simulink model "ZSM_TeslaModelS_statKreisfahrt"  (R2020b)
settings: Solver=FixedStepDiscrete  StartTime=0.0  StopTime=simtime  FixedStep=stepsize  RelTol=1e-3
undefined symbols (not defined in the file): activate_stop, activate_stop_vmax, ay_stop, ayObs, ayStiff, Bat_param, deltav_ist, DiscIntNeverNeededParam, EG_wunsch, magnitude, mu_road_LF, mu_road_LR, mu_road_RF, mu_road_RR, par_ASR, par_MDT, par_TIR, par_VEH, select_delta_h, select_M_wheel, stepsize, t, temp_betriebsstrategie, temperature_LTrange, track_left, track_right
libraries: Library_ASK x36, simulink x16, pid_lib x2, dspstat3 x2, Library_Betriebsstrategie x2, vehicle_model x2, pacejka_trans x1
(part 5 of 7)

== system ZSM_TeslaModelS_statKreisfahrt/Vehicle/Betriebsstrategie/Momentenverteilung_und_Schaltstrategie1/Limitierungen gesamt (mit MVS Limits)/Aktuatoren und Delta TV ==
  Aktuator : Constant  Value=par_MDT.AUS.akt.OD_VA
  Aktuator1 : Constant  Value=0
  Aktuator10 : Constant  Value=par_MDT.AUS.akt.TS_VA
  Aktuator11 : Constant  Value=par_MDT.AUS.akt.TS_HA
  Aktuator3 : Constant  Value=par_MDT.AUS.akt.eTV_VA
  Aktuator4 : Constant  Value=par_MDT.AUS.akt.az_VA
  Aktuator5 : Constant  Value=par_MDT.AUS.akt.OD_HA
  Aktuator6 : Constant  Value=0
  Aktuator8 : Constant  Value=par_MDT.AUS.akt.eTV_HA
  Aktuator9 : Constant  Value=par_MDT.AUS.akt.az_HA
  Limit elektrisches Überlagerungsgetriebe : Constant  Value=595
  Limit mechanisches Überlagerungsgetriebe1 : Constant  Value=595
  Limit mechanisches Überlagerungsgetriebe2 : Constant  Value=595
  Limit mechanisches Überlagerungsgetriebe3 : Constant  Value=595
  Logical Operator : Logic  Operator=NOT  AllPortsSameDT=off  OutDataTypeStr=boolean
  Logical Operator1 : Logic  Operator=NOT  AllPortsSameDT=off  OutDataTypeStr=boolean
  TV Moment pro Achse : MATLAB Function  TreatAsAtomicUnit=on
  Zuweisung Aktuatoren : MATLAB Function  TreatAsAtomicUnit=on
  Delta_T_f : Outport  VectorParamsAs1DForOutWhenUnconnected=off
  Delta_T_r : Outport  Port=2  VectorParamsAs1DForOutWhenUnconnected=off
  A_f : Outport  Port=3  VectorParamsAs1DForOutWhenUnconnected=off
  A_r : Outport  Port=4  VectorParamsAs1DForOutWhenUnconnected=off
  wires:
  Zuweisung Aktuatoren/1(a_f) -> A_f/1, TV Moment pro Achse/6(a_f)
  Aktuator9/1 -> Logical Operator1/1
  Aktuator8/1 -> Zuweisung Aktuatoren/9(A9)
  Aktuator11/1 -> Zuweisung Aktuatoren/8(A8)
  Aktuator6/1 -> Zuweisung Aktuatoren/7(A7)
  Aktuator5/1 -> Zuweisung Aktuatoren/6(A6)
  Aktuator4/1 -> Logical Operator/1
  Aktuator3/1 -> Zuweisung Aktuatoren/4(A4)
  Aktuator10/1 -> Zuweisung Aktuatoren/3(A3)
  Aktuator1/1 -> Zuweisung Aktuatoren/2(A2)
  Aktuator/1 -> Zuweisung Aktuatoren/1(A1)
  Zuweisung Aktuatoren/2(a_r) -> A_r/1, TV Moment pro Achse/7(a_r)
  TV Moment pro Achse/1(Delta_T_f) -> Delta_T_f/1
  TV Moment pro Achse/2(Delta_T_r) -> Delta_T_r/1
  Limit elektrisches Überlagerungsgetriebe/1 -> TV Moment pro Achse/1(L1)
  Limit mechanisches Überlagerungsgetriebe1/1 -> TV Moment pro Achse/2(L2)
  Limit mechanisches Überlagerungsgetriebe2/1 -> TV Moment pro Achse/3(L3)
  Limit mechanisches Überlagerungsgetriebe3/1 -> TV Moment pro Achse/4(L4)
  Logical Operator/1 -> Zuweisung Aktuatoren/5(A5)
  Logical Operator1/1 -> Zuweisung Aktuatoren/10(A10)

== system ZSM_TeslaModelS_statKreisfahrt/Vehicle/Betriebsstrategie/Momentenverteilung_und_Schaltstrategie1/Motor Limits/Limit_F_lb ==
  Raddrehzahl : Inport
  Drehmoment : Product
  Drehzahl : Product
  Getriebeuebersetzung : Constant  Value=par_MDT.VA.trans.i_gears
  Getriebewirkungsgrad : Constant  Value=par_MDT.VA.trans.wkg
  M_Reku : Lookup_n-D  NumberOfTableDimensions=1  BreakpointsForDimension1=par_MDT.VA.em.MaxGeneratorTrqCurve_w  Table=par_MDT.VA.em.MaxGeneratorTrqCurve_M  ExtrapMethod=Clip  UseLastTableValue=on  InternalRulePriority=Speed  RndMeth=Simplest  InputSameDT=on
  MinMax : MinMax  Function=max
  Rueckrechnung : Product
  Moment : Outport  VectorParamsAs1DForOutWhenUnconnected=off
  wires:
  Drehzahl/1 -> M_Reku/1
  Getriebeuebersetzung/1 -> Drehzahl/2, Drehmoment/2
  Raddrehzahl/1 -> Drehzahl/1
  M_Reku/1 -> Drehmoment/1
  Drehmoment/1 -> Rueckrechnung/1
  Rueckrechnung/1 -> MinMax/1
  Getriebewirkungsgrad/1 -> Rueckrechnung/2
  MinMax/1 -> Moment/1

== system ZSM_TeslaModelS_statKreisfahrt/Vehicle/Betriebsstrategie/Momentenverteilung_und_Schaltstrategie1/Motor Limits/Limit_F_ub ==
  Raddrehzahl : Inport
  Drehmoment : Product
  Drehzahl : Product
  Getriebeuebersetzung : Constant  Value=par_MDT.VA.trans.i_gears
  Getriebewirkungsgrad : Constant  Value=par_MDT.VA.trans.wkg
  M_Antr : Lookup_n-D  NumberOfTableDimensions=1  BreakpointsForDimension1=par_MDT.VA.em.MaxMotorTrqCurve_w  Table=par_MDT.VA.em.MaxMotorTrqCurve_M  ExtrapMethod=Clip  UseLastTableValue=on  InternalRulePriority=Speed  RndMeth=Simplest  InputSameDT=on
  MinMax : MinMax  Function=max
  Rueckrechnung : Product
  Moment : Outport  VectorParamsAs1DForOutWhenUnconnected=off
  wires:
  Drehzahl/1 -> M_Antr/1
  Getriebeuebersetzung/1 -> Drehzahl/2, Drehmoment/2
  Raddrehzahl/1 -> Drehzahl/1
  M_Antr/1 -> Drehmoment/1
  Drehmoment/1 -> Rueckrechnung/1
  Rueckrechnung/1 -> MinMax/1
  Getriebewirkungsgrad/1 -> Rueckrechnung/2
  MinMax/1 -> Moment/1

== system ZSM_TeslaModelS_statKreisfahrt/Vehicle/Betriebsstrategie/Momentenverteilung_und_Schaltstrategie1/Motor Limits/Limit_LF_lb ==
  Raddrehzahl : Inport
  Drehmoment : Product
  Drehzahl : Product
  Getriebeuebersetzung : Constant  Value=par_MDT.VA.trans.i_gears
  Getriebewirkungsgrad : Constant  Value=par_MDT.VA.trans.wkg
  M_Reku : Lookup_n-D  NumberOfTableDimensions=1  BreakpointsForDimension1=par_MDT.VA.em.MaxGeneratorTrqCurve_w  Table=par_MDT.VA.em.MaxGeneratorTrqCurve_M  ExtrapMethod=Clip  UseLastTableValue=on  InternalRulePriority=Speed  RndMeth=Simplest  InputSameDT=on
  MinMax : MinMax  Function=max
  Rueckrechnung : Product
  Moment : Outport  VectorParamsAs1DForOutWhenUnconnected=off
  wires:
  Drehzahl/1 -> M_Reku/1
  Getriebeuebersetzung/1 -> Drehzahl/2, Drehmoment/2
  Raddrehzahl/1 -> Drehzahl/1
  M_Reku/1 -> Drehmoment/1
  Drehmoment/1 -> Rueckrechnung/1
  Rueckrechnung/1 -> MinMax/1
  Getriebewirkungsgrad/1 -> Rueckrechnung/2
  MinMax/1 -> Moment/1

== system ZSM_TeslaModelS_statKreisfahrt/Vehicle/Betriebsstrategie/Momentenverteilung_und_Schaltstrategie1/Motor Limits/Limit_LF_ub ==
  Raddrehzahl : Inport
  Drehmoment : Product
  Drehzahl : Product
  Getriebeuebersetzung : Constant  Value=par_MDT.VA.trans.i_gears
  Getriebewirkungsgrad : Constant  Value=par_MDT.VA.trans.wkg
  M_Antr : Lookup_n-D  NumberOfTableDimensions=1  BreakpointsForDimension1=par_MDT.VA.em.MaxMotorTrqCurve_w  Table=par_MDT.VA.em.MaxMotorTrqCurve_M  ExtrapMethod=Clip  UseLastTableValue=on  InternalRulePriority=Speed  RndMeth=Simplest  InputSameDT=on
  MinMax : MinMax  Function=max
  Rueckrechnung : Product
  Moment : Outport  VectorParamsAs1DForOutWhenUnconnected=off
  wires:
  Drehzahl/1 -> M_Antr/1
  Getriebeuebersetzung/1 -> Drehzahl/2, Drehmoment/2
  Raddrehzahl/1 -> Drehzahl/1
  M_Antr/1 -> Drehmoment/1
  Drehmoment/1 -> Rueckrechnung/1
  Rueckrechnung/1 -> MinMax/1
  Getriebewirkungsgrad/1 -> Rueckrechnung/2
  MinMax/1 -> Moment/1

== system ZSM_TeslaModelS_statKreisfahrt/Vehicle/Betriebsstrategie/Momentenverteilung_und_Schaltstrategie1/Motor Limits/Limit_LR_lb ==
  Raddrehzahl : Inport
  Drehmoment : Product
  Drehzahl : Product
  Getriebeuebersetzung : Constant  Value=par_MDT.HA.trans.i_gears
  Getriebewirkungsgrad : Constant  Value=par_MDT.HA.trans.wkg
  M_Reku : Lookup_n-D  NumberOfTableDimensions=1  BreakpointsForDimension1=par_MDT.HA.em.MaxGeneratorTrqCurve_w  Table=par_MDT.HA.em.MaxGeneratorTrqCurve_M  ExtrapMethod=Clip  UseLastTableValue=on  InternalRulePriority=Speed  RndMeth=Simplest  InputSameDT=on
  MinMax : MinMax  Function=max
  Rueckrechnung : Product
  Moment : Outport  VectorParamsAs1DForOutWhenUnconnected=off
  wires:
  Drehzahl/1 -> M_Reku/1
  Getriebeuebersetzung/1 -> Drehzahl/2, Drehmoment/2
  Raddrehzahl/1 -> Drehzahl/1
  M_Reku/1 -> Drehmoment/1
  Drehmoment/1 -> Rueckrechnung/1
  Rueckrechnung/1 -> MinMax/1
  Getriebewirkungsgrad/1 -> Rueckrechnung/2
  MinMax/1 -> Moment/1

== system ZSM_TeslaModelS_statKreisfahrt/Vehicle/Betriebsstrategie/Momentenverteilung_und_Schaltstrategie1/Motor Limits/Limit_LR_ub ==
  Raddrehzahl : Inport
  Drehmoment : Product
  Drehzahl : Product
  Getriebeuebersetzung : Constant  Value=par_MDT.HA.trans.i_gears
  Getriebewirkungsgrad : Constant  Value=par_MDT.HA.trans.wkg
  M_Antr : Lookup_n-D  NumberOfTableDimensions=1  BreakpointsForDimension1=par_MDT.HA.em.MaxMotorTrqCurve_w  Table=par_MDT.HA.em.MaxMotorTrqCurve_M  ExtrapMethod=Clip  UseLastTableValue=on  InternalRulePriority=Speed  RndMeth=Simplest  InputSameDT=on
  MinMax : MinMax  Function=max
  Rueckrechnung : Product
  Moment : Outport  VectorParamsAs1DForOutWhenUnconnected=off
  wires:
  Drehzahl/1 -> M_Antr/1
  Getriebeuebersetzung/1 -> Drehzahl/2, Drehmoment/2
  Raddrehzahl/1 -> Drehzahl/1
  M_Antr/1 -> Drehmoment/1
  Drehmoment/1 -> Rueckrechnung/1
  Rueckrechnung/1 -> MinMax/1
  Getriebewirkungsgrad/1 -> Rueckrechnung/2
  MinMax/1 -> Moment/1

== system ZSM_TeslaModelS_statKreisfahrt/Vehicle/Betriebsstrategie/Momentenverteilung_und_Schaltstrategie1/Motor Limits/Limit_RF_lb ==
  Raddrehzahl : Inport
  Drehmoment : Product
  Drehzahl : Product
  Getriebeuebersetzung : Constant  Value=par_MDT.VA.trans.i_gears
  Getriebewirkungsgrad : Constant  Value=par_MDT.VA.trans.wkg
  M_Reku : Lookup_n-D  NumberOfTableDimensions=1  BreakpointsForDimension1=par_MDT.VA.em.MaxGeneratorTrqCurve_w  Table=par_MDT.VA.em.MaxGeneratorTrqCurve_M  ExtrapMethod=Clip  UseLastTableValue=on  InternalRulePriority=Speed  RndMeth=Simplest  InputSameDT=on
  MinMax : MinMax  Function=max
  Rueckrechnung : Product
  Moment : Outport  VectorParamsAs1DForOutWhenUnconnected=off
  wires:
  Drehzahl/1 -> M_Reku/1
  Getriebeuebersetzung/1 -> Drehzahl/2, Drehmoment/2
  Raddrehzahl/1 -> Drehzahl/1
  M_Reku/1 -> Drehmoment/1
  Drehmoment/1 -> Rueckrechnung/1
  Rueckrechnung/1 -> MinMax/1
  Getriebewirkungsgrad/1 -> Rueckrechnung/2
  MinMax/1 -> Moment/1

== system ZSM_TeslaModelS_statKreisfahrt/Vehicle/Betriebsstrategie/Momentenverteilung_und_Schaltstrategie1/Motor Limits/Limit_RF_ub ==
  Raddrehzahl : Inport
  Drehmoment : Product
  Drehzahl : Product
  Getriebeuebersetzung : Constant  Value=par_MDT.VA.trans.i_gears
  Getriebewirkungsgrad : Constant  Value=par_MDT.VA.trans.wkg
  M_Antr : Lookup_n-D  NumberOfTableDimensions=1  BreakpointsForDimension1=par_MDT.VA.em.MaxMotorTrqCurve_w  Table=par_MDT.VA.em.MaxMotorTrqCurve_M  ExtrapMethod=Clip  UseLastTableValue=on  InternalRulePriority=Speed  RndMeth=Simplest  InputSameDT=on
  MinMax : MinMax  Function=max
  Rueckrechnung : Product
  Moment : Outport  VectorParamsAs1DForOutWhenUnconnected=off
  wires:
  Drehzahl/1 -> M_Antr/1
  Getriebeuebersetzung/1 -> Drehzahl/2, Drehmoment/2
  Raddrehzahl/1 -> Drehzahl/1
  M_Antr/1 -> Drehmoment/1
  Drehmoment/1 -> Rueckrechnung/1
  Rueckrechnung/1 -> MinMax/1
  Getriebewirkungsgrad/1 -> Rueckrechnung/2
  MinMax/1 -> Moment/1

== system ZSM_TeslaModelS_statKreisfahrt/Vehicle/Betriebsstrategie/Momentenverteilung_und_Schaltstrategie1/Motor Limits/Limit_RR_lb ==
  Raddrehzahl : Inport
  Drehmoment : Product
  Drehzahl : Product
  Getriebeuebersetzung : Constant  Value=par_MDT.HA.trans.i_gears
  Getriebewirkungsgrad : Constant  Value=par_MDT.HA.trans.wkg
  M_Reku : Lookup_n-D  NumberOfTableDimensions=1  BreakpointsForDimension1=par_MDT.HA.em.MaxGeneratorTrqCurve_w  Table=par_MDT.HA.em.MaxGeneratorTrqCurve_M  ExtrapMethod=Clip  UseLastTableValue=on  InternalRulePriority=Speed  RndMeth=Simplest  InputSameDT=on
  MinMax : MinMax  Function=max
  Rueckrechnung : Product
  Moment : Outport  VectorParamsAs1DForOutWhenUnconnected=off
  wires:
  Drehzahl/1 -> M_Reku/1
  Getriebeuebersetzung/1 -> Drehzahl/2, Drehmoment/2
  Raddrehzahl/1 -> Drehzahl/1
  M_Reku/1 -> Drehmoment/1
  Drehmoment/1 -> Rueckrechnung/1
  Rueckrechnung/1 -> MinMax/1
  Getriebewirkungsgrad/1 -> Rueckrechnung/2
  MinMax/1 -> Moment/1

== system ZSM_TeslaModelS_statKreisfahrt/Vehicle/Betriebsstrategie/Momentenverteilung_und_Schaltstrategie1/Motor Limits/Limit_RR_ub ==
  Raddrehzahl : Inport
  Drehmoment : Product
  Drehzahl : Product
  Getriebeuebersetzung : Constant  Value=par_MDT.HA.trans.i_gears
  Getriebewirkungsgrad : Constant  Value=par_MDT.HA.trans.wkg
  M_Antr : Lookup_n-D  NumberOfTableDimensions=1  BreakpointsForDimension1=par_MDT.HA.em.MaxMotorTrqCurve_w  Table=par_MDT.HA.em.MaxMotorTrqCurve_M  ExtrapMethod=Clip  UseLastTableValue=on  InternalRulePriority=Speed  RndMeth=Simplest  InputSameDT=on
  MinMax : MinMax  Function=max
  Rueckrechnung : Product
  Moment : Outport  VectorParamsAs1DForOutWhenUnconnected=off
  wires:
  Drehzahl/1 -> M_Antr/1
  Getriebeuebersetzung/1 -> Drehzahl/2, Drehmoment/2
  Raddrehzahl/1 -> Drehzahl/1
  M_Antr/1 -> Drehmoment/1
  Drehmoment/1 -> Rueckrechnung/1
  Rueckrechnung/1 -> MinMax/1
  Getriebewirkungsgrad/1 -> Rueckrechnung/2
  MinMax/1 -> Moment/1

== system ZSM_TeslaModelS_statKreisfahrt/Vehicle/Betriebsstrategie/Momentenverteilung_und_Schaltstrategie1/Motor Limits/Limit_R_lb ==
  Raddrehzahl : Inport
  Drehmoment : Product
  Drehzahl : Product
  Getriebeuebersetzung : Constant  Value=par_MDT.HA.trans.i_gears
  Getriebewirkungsgrad : Constant  Value=par_MDT.HA.trans.wkg
  M_Reku : Lookup_n-D  NumberOfTableDimensions=1  BreakpointsForDimension1=par_MDT.HA.em.MaxGeneratorTrqCurve_w  Table=par_MDT.HA.em.MaxGeneratorTrqCurve_M  ExtrapMethod=Clip  UseLastTableValue=on  InternalRulePriority=Speed  RndMeth=Simplest  InputSameDT=on
  MinMax : MinMax  Function=max
  Rueckrechnung : Product
  Moment : Outport  VectorParamsAs1DForOutWhenUnconnected=off
  wires:
  Drehzahl/1 -> M_Reku/1
  Getriebeuebersetzung/1 -> Drehzahl/2, Drehmoment/2
  Raddrehzahl/1 -> Drehzahl/1
  M_Reku/1 -> Drehmoment/1
  Drehmoment/1 -> Rueckrechnung/1
  Rueckrechnung/1 -> MinMax/1
  Getriebewirkungsgrad/1 -> Rueckrechnung/2
  MinMax/1 -> Moment/1

== system ZSM_TeslaModelS_statKreisfahrt/Vehicle/Betriebsstrategie/Momentenverteilung_und_Schaltstrategie1/Motor Limits/Limit_R_ub ==
  Raddrehzahl : Inport
  Drehmoment : Product
  Drehzahl : Product
  Getriebeuebersetzung : Constant  Value=par_MDT.HA.trans.i_gears
  Getriebewirkungsgrad : Constant  Value=par_MDT.HA.trans.wkg
  M_Antr : Lookup_n-D  NumberOfTableDimensions=1  BreakpointsForDimension1=par_MDT.HA.em.MaxMotorTrqCurve_w  Table=par_MDT.HA.em.MaxMotorTrqCurve_M  ExtrapMethod=Clip  UseLastTableValue=on  InternalRulePriority=Speed  RndMeth=Simplest  InputSameDT=on
  MinMax : MinMax  Function=max
  Rueckrechnung : Product
  Moment : Outport  VectorParamsAs1DForOutWhenUnconnected=off
  wires:
  Drehzahl/1 -> M_Antr/1
  Getriebeuebersetzung/1 -> Drehzahl/2, Drehmoment/2
  Raddrehzahl/1 -> Drehzahl/1
  M_Antr/1 -> Drehmoment/1
  Drehmoment/1 -> Rueckrechnung/1
  Rueckrechnung/1 -> MinMax/1
  Getriebewirkungsgrad/1 -> Rueckrechnung/2
  MinMax/1 -> Moment/1

== system ZSM_TeslaModelS_statKreisfahrt/Vehicle/Betriebsstrategie/Momentenverteilung_und_Schaltstrategie1/Radmomentenaufteilung (Effizienz)/Axle activator ==
  Add4 : Sum
  Add6 : Sum
  Constant3 : Constant  Value=par_MDT.AUS.akt.az_VA
  Constant4 : Constant  Value=par_MDT.AUS.akt.az_HA
  Constant5 : Constant  Value=par_MDT.AUS.akt.rn_HA
  Constant6 : Constant  Value=par_MDT.AUS.akt.rn_VA
  VA : Outport  VectorParamsAs1DForOutWhenUnconnected=off
  HA : Outport  Port=2  VectorParamsAs1DForOutWhenUnconnected=off
  wires:
  Add4/1 -> VA/1
  Constant6/1 -> Add4/2
  Constant3/1 -> Add4/1
  Constant5/1 -> Add6/2
  Add6/1 -> HA/1
  Constant4/1 -> Add6/1

== system ZSM_TeslaModelS_statKreisfahrt/Vehicle/Betriebsstrategie/Momentenverteilung_und_Schaltstrategie1/Radmomentenaufteilung (Effizienz)/Limits ermitteln ==
  M_VA_max : Inport
  M_VA_min : Inport  Port=2
  M_HA_max : Inport  Port=3
  M_HA_min : Inport  Port=4
  M_wheel_in : Inport  Port=5
  Abs{,1..3} (4 alike) : Abs
  Add : Sum
  Axle activator : Subsystem
  Falls M_wheel kleiner als M_VA_pot : Subsystem
  Gain : Gain  Gain=0.98
  Logical Operator : Logic  Operator=XOR  AllPortsSameDT=off  OutDataTypeStr=boolean
  Min : MinMax  Inputs=2
  Product : Product
  Relational Operator : RelationalOperator  Operator=<  OutDataTypeStr=boolean  RndMeth=Simplest
  Sign : Signum
  Switch{,1..4} (5 alike) : Switch  Criteria=u2 > Threshold
  M_VA_pot : Outport  VectorParamsAs1DForOutWhenUnconnected=off
  M_HA_pot : Outport  Port=2  VectorParamsAs1DForOutWhenUnconnected=off
  M_wheel_out : Outport  Port=3  VectorParamsAs1DForOutWhenUnconnected=off
  Major index : Outport  Port=4  VectorParamsAs1DForOutWhenUnconnected=off
  Rekuindex : Outport  Port=5  VectorParamsAs1DForOutWhenUnconnected=off
  wires:
  M_wheel_in/1 -> Sign/1, Falls M_wheel kleiner als M_VA_pot/2(M_wheel)
  M_HA_max/1 -> Switch1/1
  M_HA_min/1 -> Switch1/3
  M_VA_max/1 -> Switch2/1
  M_VA_min/1 -> Switch2/3
  Switch2/1 -> Switch3/3, Add/1, Abs2/1, Falls M_wheel kleiner als M_VA_pot/1(M_VA_pot_in)
  Switch3/1 -> M_VA_pot/1
  Abs1/1 -> Min/2
  Min/1 -> Product/2
  Switch/1 -> M_HA_pot/1
  Sign/1 -> Switch2/2, Product/1, Rekuindex/1, Falls M_wheel kleiner als M_VA_pot/3(Rekuindex), Switch1/2  "Rekuindex"
  Falls M_wheel kleiner als M_VA_pot/2(M_wheel_out) -> Abs1/1
  Abs/1 -> Min/1
  Add/1 -> Abs/1
  Product/1 -> M_wheel_out/1
  Switch1/1 -> Add/2, Switch/1, Abs3/1, Falls M_wheel kleiner als M_VA_pot/4(M_HA_pot_in)
  Falls M_wheel kleiner als M_VA_pot/1(M_VA_pot_out) -> Switch3/1
  Falls M_wheel kleiner als M_VA_pot/3(M_HA_pot_out) -> Switch/3
  Switch4/1 -> Switch/2, Major index/1, Switch3/2
  Axle activator/2(HA) -> Logical Operator/2
  Axle activator/1(VA) -> Logical Operator/1
  Relational Operator/1 -> Switch4/3
  Logical Operator/1 -> Switch4/2, Switch4/1
  Gain/1 -> Relational Operator/1
  Abs2/1 -> Gain/1
  Abs3/1 -> Relational Operator/2

== system ZSM_TeslaModelS_statKreisfahrt/Vehicle/Betriebsstrategie/Momentenverteilung_und_Schaltstrategie1/Radmomentenaufteilung (Effizienz)/Momentenrückführung und Motormomentberechnung ==
  M_VA_in : Inport
  M_VA_pot : Inport  Port=2
  M_HA_in : Inport  Port=3
  M_HA_pot : Inport  Port=4
  Major_index : Inport  Port=5
  Rekuperationsindex : Inport  Port=6
  i_VA : Inport  Port=7
  i_HA : Inport  Port=8
  Divide1 : Product  Inputs=/*
  Divide2 : Product  Inputs=/*
  Divide5 : Product  Inputs=*/
  Divide6 : Product  Inputs=*/
  Getriebewirkungsgradberechnung Hinterachse : Subsystem
  Getriebewirkungsgradberechnung Vorderachse : Subsystem
  Logical Operator : Logic  Operator=NOT  AllPortsSameDT=off  OutDataTypeStr=boolean
  Subsystem : Subsystem
  Subsystem1 : Subsystem
  Switch1 : Switch  Criteria=u2 > Threshold
  Switch2 : Switch  Criteria=u2 > Threshold
  M_VA_mot : Outport  VectorParamsAs1DForOutWhenUnconnected=off
  M_VA : Outport  Port=2  VectorParamsAs1DForOutWhenUnconnected=off
  Rekuindex : Outport  Port=3  VectorParamsAs1DForOutWhenUnconnected=off
  M_HA_mot : Outport  Port=4  VectorParamsAs1DForOutWhenUnconnected=off
  M_HA : Outport  Port=5  VectorParamsAs1DForOutWhenUnconnected=off
  wires:
  M_VA_in/1 -> Divide6/1
  i_VA/1 -> Divide6/2, Divide2/1
  Divide6/1 -> M_VA/1, Getriebewirkungsgradberechnung Vorderachse/1(M_VA_mot)  "M_VA"
  Rekuperationsindex/1 -> Getriebewirkungsgradberechnung Hinterachse/1(Rekuindex), Rekuindex/1, Getriebewirkungsgradberechnung Vorderachse/2(Rekuindex)
  M_HA_in/1 -> Divide1/2
  i_HA/1 -> Divide1/1, Divide5/2
  Divide1/1 -> M_HA/1, Getriebewirkungsgradberechnung Hinterachse/2(M_HA_mot)
  M_HA_pot/1 -> Divide5/1
  M_VA_pot/1 -> Divide2/2
  Getriebewirkungsgradberechnung Vorderachse/1(WKG_GTR_VA) -> Subsystem/2(M_VA_mot_in), Switch1/1  "M_VA_mot"
  Divide2/1 -> Subsystem/1(M_VA_pot)
  Switch1/1 -> M_VA_mot/1
  Divide5/1 -> Subsystem1/1(M_HA_pot)
  Getriebewirkungsgradberechnung Hinterachse/1(WKG_GTR_HA) -> Subsystem1/2(M_HA_mot_in), Switch2/3
  Switch2/1 -> M_HA_mot/1
  Subsystem/1(M_VA_mot_out) -> Switch1/3
  Subsystem1/1(M_HA_mot_out) -> Switch2/1
  Major_index/1 -> Logical Operator/1, Subsystem1/Enable, Switch2/2, Switch1/2
  Logical Operator/1 -> Subsystem/Enable

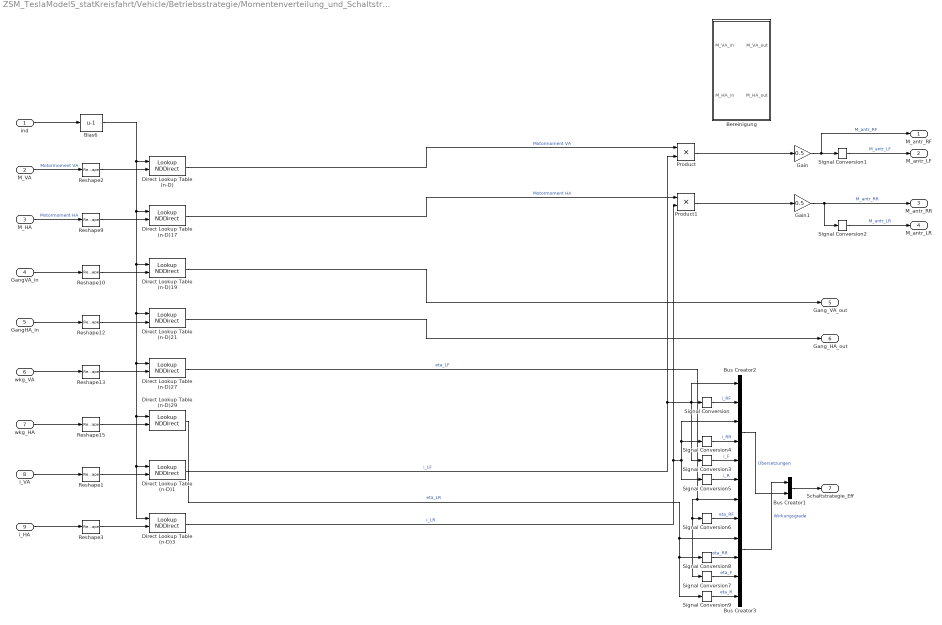
== system ZSM_TeslaModelS_statKreisfahrt/Vehicle/Betriebsstrategie/Momentenverteilung_und_Schaltstrategie1/Radmomentenaufteilung (Effizienz)/Optimierung und Schaltstrategie ==
  ind : Inport
  M_VA : Inport  Port=2
  M_HA : Inport  Port=3
  GangVA_in : Inport  Port=4
  GangHA_in : Inport  Port=5
  wkg_VA : Inport  Port=6
  wkg_HA : Inport  Port=7
  i_VA : Inport  Port=8
  i_HA : Inport  Port=9
  Bereinigung : Subsystem
  Bias6 : Bias  Bias=-1
  Bus Creator1 : BusCreator  Inputs=2
  Bus Creator2 : BusCreator  Inputs=6
  Bus Creator3 : BusCreator  Inputs=6
  Direct Lookup Table (n-D){,1,3,17,19,21,27,29} (8 alike) : LookupNDDirect  NumberOfTableDimensions=1  TableIsInput=on
  Gain : Gain  Gain=0.5
  Gain1 : Gain  Gain=0.5
  Product : Product
  Product1 : Product
  Reshape{1..3,9..10,12..13,15} (8 alike) : Reshape
  Signal Conversion{,1..9} (10 alike) : SignalConversion  OverrideOpt=off
  M_antr_RF : Outport  VectorParamsAs1DForOutWhenUnconnected=off
  M_antr_LF : Outport  Port=2  VectorParamsAs1DForOutWhenUnconnected=off
  M_antr_RR : Outport  Port=3  VectorParamsAs1DForOutWhenUnconnected=off
  M_antr_LR : Outport  Port=4  VectorParamsAs1DForOutWhenUnconnected=off
  Gang_VA_out : Outport  Port=5  VectorParamsAs1DForOutWhenUnconnected=off
  Gang_HA_out : Outport  Port=6  VectorParamsAs1DForOutWhenUnconnected=off
  Schaltstrategie_Eff : Outport  Port=7  VectorParamsAs1DForOutWhenUnconnected=off
  wires:
  Gain/1 -> Signal Conversion1/1, M_antr_RF/1  "M_antr_RF"
  Gain1/1 -> Signal Conversion2/1, M_antr_RR/1  "M_antr_RR"
  Signal Conversion1/1 -> M_antr_LF/1  "M_antr_LF"
  Signal Conversion2/1 -> M_antr_LR/1  "M_antr_LR"
  Direct Lookup Table (n-D)1/1 -> Product/2, Signal Conversion/1, Bus Creator2/1, Signal Conversion3/1  "i_LF"
  Direct Lookup Table (n-D)3/1 -> Product1/2, Signal Conversion5/1, Signal Conversion4/1, Bus Creator2/3  "i_LR"
  Direct Lookup Table (n-D)29/1 -> Signal Conversion9/1, Signal Conversion8/1, Bus Creator3/3  "eta_LR"
  Direct Lookup Table (n-D)27/1 -> Signal Conversion7/1, Signal Conversion6/1, Bus Creator3/1  "eta_LF"
  Bus Creator1/1 -> Schaltstrategie_Eff/1
  Bus Creator3/1 -> Bus Creator1/1  "Wirkungsgrade"
  Bus Creator2/1 -> Bus Creator1/2  "Übersetzungen"
  Signal Conversion/1 -> Bus Creator2/2  "i_RF"
  Signal Conversion3/1 -> Bus Creator2/5  "i_F"
  Signal Conversion4/1 -> Bus Creator2/4  "i_RR"
  Signal Conversion5/1 -> Bus Creator2/6  "i_R"
  Signal Conversion6/1 -> Bus Creator3/2  "eta_RF"
  Signal Conversion7/1 -> Bus Creator3/5  "eta_F"
  Signal Conversion8/1 -> Bus Creator3/4  "eta_RR"
  Signal Conversion9/1 -> Bus Creator3/6  "eta_R"
  Direct Lookup Table (n-D)19/1 -> Gang_VA_out/1
  Direct Lookup Table (n-D)21/1 -> Gang_HA_out/1
  ind/1 -> Bias6/1
  Reshape2/1 -> Direct Lookup Table (n-D)/2
  Reshape9/1 -> Direct Lookup Table (n-D)17/2
  Reshape10/1 -> Direct Lookup Table (n-D)19/2
  Reshape12/1 -> Direct Lookup Table (n-D)21/2
  Reshape13/1 -> Direct Lookup Table (n-D)27/2
  GangVA_in/1 -> Reshape10/1
  GangHA_in/1 -> Reshape12/1
  Reshape15/1 -> Direct Lookup Table (n-D)29/2
  wkg_VA/1 -> Reshape13/1
  wkg_HA/1 -> Reshape15/1
  Direct Lookup Table (n-D)/1 -> Product/1  "Motormoment VA"
  Direct Lookup Table (n-D)17/1 -> Product1/1  "Motormoment HA"
  M_HA/1 -> Reshape9/1  "Motormoment HA"
  M_VA/1 -> Reshape2/1  "Motormoment VA"
  Reshape1/1 -> Direct Lookup Table (n-D)1/2
  Reshape3/1 -> Direct Lookup Table (n-D)3/2
  i_VA/1 -> Reshape1/1
  i_HA/1 -> Reshape3/1
  Product1/1 -> Gain1/1
  Product/1 -> Gain/1
  Bias6/1 -> Direct Lookup Table (n-D)17/1, Direct Lookup Table (n-D)19/1, Direct Lookup Table (n-D)21/1, Direct Lookup Table (n-D)27/1, Direct Lookup Table (n-D)1/1, Direct Lookup Table (n-D)3/1, Direct Lookup Table (n-D)29/1, Direct Lookup Table (n-D)/1

== system ZSM_TeslaModelS_statKreisfahrt/Vehicle/Betriebsstrategie/Momentenverteilung_und_Schaltstrategie1/Radmomentenaufteilung (Effizienz)/Subsystem ==
  n_mot_VA : Inport
  M_Achs_EM_VA : Inport  Port=2
  Rekuindex : Inport  Port=3
  Enable : EnablePort
  Inverter Power Input einer Achse : Library_Betriebsstrategie/Inverter Power Input  einer Achse  U_RMS=par_MDT.VA.em.U_RMS  az=par_MDT.AUS.akt.az_VA  Powerfactor_map=par_MDT.VA.inv.Powerfactor_map  torque=par_MDT.VA.inv.torque  speed=par_MDT.VA.inv.speed  efficiency_map_LE=par_MDT.VA.inv.efficiency_map.efficiency_map_LE  current=par_MDT.VA.inv.current  voltage=par_MDT.VA.inv.voltage  powerfactor=par_MDT.VA.inv.powerfactor  MotorEffMap3D=par_MDT.VA.em.MotorEffMap3D  MotorEffMap3D_w=par_MDT.VA.em.MotorEffMap3D_w  MotorEffMap3D_M=par_MDT.VA.em.MotorEffMap3D_M  GeneratorEffMap3D=par_MDT.VA.em.GeneratorEffMap3D  GeneratorEffMap3D_w=par_MDT.VA.em.GeneratorEffMap3D_w  GeneratorEffMap3D_M=par_MDT.VA.em.GeneratorEffMap3D_M
  P_achs_VA : Outport  VectorParamsAs1DForOutWhenUnconnected=off
  wires:
  n_mot_VA/1 -> Inverter Power Input einer Achse/1
  M_Achs_EM_VA/1 -> Inverter Power Input einer Achse/2
  Inverter Power Input einer Achse/1 -> P_achs_VA/1
  Rekuindex/1 -> Inverter Power Input einer Achse/3

== system ZSM_TeslaModelS_statKreisfahrt/Vehicle/Betriebsstrategie/Momentenverteilung_und_Schaltstrategie1/Radmomentenaufteilung (Effizienz)/Subsystem1 ==
  Rekuindex : Inport
  n_mot_HA : Inport  Port=2
  M_Achs_EM_HA : Inport  Port=3
  Enable : EnablePort
  Inverter Power Input einer Achse1 : Library_Betriebsstrategie/Inverter Power Input  einer Achse  U_RMS=par_MDT.HA.em.U_RMS  az=par_MDT.AUS.akt.az_HA  Powerfactor_map=par_MDT.HA.inv.Powerfactor_map  torque=par_MDT.HA.inv.torque  speed=par_MDT.HA.inv.speed  efficiency_map_LE=par_MDT.HA.inv.efficiency_map.efficiency_map_LE  current=par_MDT.HA.inv.current  voltage=par_MDT.HA.inv.voltage  powerfactor=par_MDT.HA.inv.powerfactor  MotorEffMap3D=par_MDT.HA.em.MotorEffMap3D  MotorEffMap3D_w=par_MDT.HA.em.MotorEffMap3D_w  MotorEffMap3D_M=par_MDT.HA.em.MotorEffMap3D_M  GeneratorEffMap3D=par_MDT.HA.em.GeneratorEffMap3D  GeneratorEffMap3D_w=par_MDT.HA.em.GeneratorEffMap3D_w  GeneratorEffMap3D_M=par_MDT.HA.em.GeneratorEffMap3D_M
  P_achs_HA : Outport  VectorParamsAs1DForOutWhenUnconnected=off
  wires:
  n_mot_HA/1 -> Inverter Power Input einer Achse1/1
  Inverter Power Input einer Achse1/1 -> P_achs_HA/1
  M_Achs_EM_HA/1 -> Inverter Power Input einer Achse1/2
  Rekuindex/1 -> Inverter Power Input einer Achse1/3

== system ZSM_TeslaModelS_statKreisfahrt/Vehicle/Betriebsstrategie/Momentenverteilung_und_Schaltstrategie1/Radmomentenaufteilung (Effizienz)/Torque shift damper ==
  P_achs : Inport
  M_target : Inport  Port=2
  Axle activator : Subsystem
  Logical Operator : Logic  Operator=NOT  AllPortsSameDT=off  OutDataTypeStr=boolean
  Optimierung_damped_AWD : Subsystem
  Optimierung_eine_achs : Subsystem
  Product1 : Product
  Switch : Switch  Criteria=u2 > Threshold
  Switch1 : Switch  Criteria=u2 > Threshold
  P_opt : Outport  VectorParamsAs1DForOutWhenUnconnected=off
  ind : Outport  Port=2  VectorParamsAs1DForOutWhenUnconnected=off
  Akt : Outport  Port=3  VectorParamsAs1DForOutWhenUnconnected=off
  wires:
  M_target/1 -> Optimierung_eine_achs/2(M_target), Optimierung_damped_AWD/2(M_target)
  Switch/1 -> P_opt/1
  Switch1/1 -> ind/1
  Optimierung_damped_AWD/2(ind) -> Switch1/1
  Optimierung_damped_AWD/1(P_opt) -> Switch/1
  Product1/1 -> Switch1/2, Switch/2, Akt/1, Logical Operator/1, Optimierung_damped_AWD/Enable
  P_achs/1 -> Optimierung_eine_achs/1(P_achs), Optimierung_damped_AWD/1(P_achs)
  Optimierung_eine_achs/2("ind ") -> Switch1/3
  Optimierung_eine_achs/1("P_opt ") -> Switch/3
  Logical Operator/1 -> Optimierung_eine_achs/Enable
  Axle activator/1(VA) -> Optimierung_eine_achs/3(Akt_VA), Product1/1
  Axle activator/2(HA) -> Product1/2, Optimierung_eine_achs/4(Akt_HA)

== system ZSM_TeslaModelS_statKreisfahrt/Vehicle/Betriebsstrategie/Momentenverteilung_und_Schaltstrategie1/Radmomentenaufteilung (Effizienz)/Torque variation limiter ==
  note: Luca Mantovani, 05.9.18
      | This blocks limits torque variation to a certain rate, when the smart torque allocation system is enabled, and compensate it to still obtain the overall vehicle torque required
  Akt : Inport
  M_wheel_in : Inport  Port=2
  M_antr_RF : Inport  Port=3
  M_antr_LF : Inport  Port=4
  M_antr_RR : Inport  Port=5
  M_antr_LR : Inport  Port=6
  Add{,1..3} (4 alike) : Sum
  Add5 : Sum  Inputs=++++
  Constant : Constant  Value=0
  Gain : Gain  Gain=0.25
  Rate Limiter{1..4} (4 alike) : RateLimiter  RisingSlewLimit=800  FallingSlewLimit=-800  SampleTimeMode=inherited
  Subtract : Sum  Inputs=+-
  Switch{,1..4} (5 alike) : Switch  Criteria=u2 > Threshold
  M_antr_korr_RF : Outport  VectorParamsAs1DForOutWhenUnconnected=off
  M_antr_korr_LF : Outport  Port=2  VectorParamsAs1DForOutWhenUnconnected=off
  M_antr_korr_RR : Outport  Port=3  VectorParamsAs1DForOutWhenUnconnected=off
  M_antr_korr_LR : Outport  Port=4  VectorParamsAs1DForOutWhenUnconnected=off
  wires:
  Switch3/1 -> Add2/1, Add5/2
  Switch1/1 -> Add/1, Add5/4
  Switch2/1 -> Add1/1, Add5/3
  Switch4/1 -> Add5/1, Add3/1
  M_antr_LR/1 -> Rate Limiter4/1, Switch4/3
  M_antr_RF/1 -> Switch1/3, Rate Limiter1/1
  M_antr_LF/1 -> Rate Limiter2/1, Switch2/3
  M_antr_RR/1 -> Rate Limiter3/1, Switch3/3
  Subtract/1 -> Gain/1
  Add5/1 -> Subtract/2
  M_wheel_in/1 -> Subtract/1
  Switch/1 -> Add/2, Add1/2, Add2/2, Add3/2
  Add/1 -> M_antr_korr_RF/1  "M_antr_RF"
  Add1/1 -> M_antr_korr_LF/1  "M_antr_LF"
  Add3/1 -> M_antr_korr_LR/1  "M_antr_LR"
  Add2/1 -> M_antr_korr_RR/1  "M_antr_RR"
  Gain/1 -> Switch/1
  Constant/1 -> Switch/3
  Akt/1 -> Switch1/2, Switch2/2, Switch3/2, Switch/2, Switch4/2
  Rate Limiter1/1 -> Switch1/1
  Rate Limiter2/1 -> Switch2/1
  Rate Limiter3/1 -> Switch3/1
  Rate Limiter4/1 -> Switch4/1

== system ZSM_TeslaModelS_statKreisfahrt/Vehicle/Betriebsstrategie/Momentenverteilung_und_Schaltstrategie1/Radmomentenaufteilung (Effizienz)/Umrechnung auf Motordrehzahl ==
  note: Absolut weil die Kennfelder keine negative Drehzahlen abbilden
  n_VA : Inport
  n_HA : Inport  Port=2
  Abs : Abs
  Abs1 : Abs
  Constant : Constant  Value=ones(par_MDT.VA.trans.n_gears*par_MDT.HA.trans.n_gears,par_VEH.dt.ecu.Vektorlaenge)  VectorParams1D=off
  Constant1 : Constant  Value=par_VEH.dt.ecu.Uebersetzungen_HA
  Constant2 : Constant  Value=par_VEH.dt.ecu.Uebersetzungen_VA
  Divide : Product  Inputs=**
  Divide3 : Product  Inputs=**
  Product7 : Product
  Product8 : Product
  n_VA_mot : Outport  VectorParamsAs1DForOutWhenUnconnected=off
  n_HA_mot : Outport  Port=2  VectorParamsAs1DForOutWhenUnconnected=off
  wires:
  Constant/1 -> Product8/2, Product7/2
  Product7/1 -> Divide/2
  n_HA/1 -> Product8/1
  Product8/1 -> Divide3/1
  n_VA/1 -> Product7/1
  Divide3/1 -> Abs1/1
  Constant2/1 -> Divide/1
  Constant1/1 -> Divide3/2
  Divide/1 -> Abs/1
  Abs/1 -> n_VA_mot/1
  Abs1/1 -> n_HA_mot/1

== system ZSM_TeslaModelS_statKreisfahrt/Vehicle/Betriebsstrategie/Momentenverteilung_und_Schaltstrategie1/Radmomentenaufteilung (Effizienz)/Umverteilung nur 1% pro Zeitschritt ==
  ind_unlim : Inport
  Add : Sum  Inputs=3
  Bias1 : Bias  Bias=par_VEH.dt.ecu.n_Schaltkombinationen
  Bias2 : Bias  Bias=-par_VEH.dt.ecu.n_Schaltkombinationen
  Constant : Constant  Value=2
  Constant1 : Constant  Value=0
  Constant2 : Constant
  Constant3 : Constant  Value=0
  Constant4 : Constant  Value=3
  Constant5 : Constant  Value=0
  Memory : Memory
  Multiport Switch : MultiPortSwitch  DataPortOrder=Specify indices
  Relational Operator : RelationalOperator  Operator=>  OutDataTypeStr=boolean  RndMeth=Nearest
  Relational Operator1 : RelationalOperator  Operator=<  OutDataTypeStr=boolean  RndMeth=Nearest
  Relational Operator2 : RelationalOperator  Operator===  OutDataTypeStr=boolean  RndMeth=Nearest
  Switch : Switch  Criteria=u2 > Threshold
  Switch1 : Switch  Criteria=u2 > Threshold
  Switch2 : Switch  Criteria=u2 > Threshold
  ind_lim : Outport  VectorParamsAs1DForOutWhenUnconnected=off
  wires:
  ind_unlim/1 -> Relational Operator/1, Relational Operator1/1, Relational Operator2/1
  Multiport Switch/1 -> Memory/1, ind_lim/1
  Memory/1 -> Bias2/1, Multiport Switch/3, Bias1/1, Relational Operator/2, Relational Operator2/2, Relational Operator1/2
  Relational Operator2/1 -> Switch/2
  Bias1/1 -> Multiport Switch/4
  Bias2/1 -> Multiport Switch/2
  Constant/1 -> Switch/1
  Constant1/1 -> Switch/3
  Relational Operator1/1 -> Switch1/2
  Constant2/1 -> Switch1/1
  Constant3/1 -> Switch1/3
  Relational Operator/1 -> Switch2/2
  Constant4/1 -> Switch2/1
  Constant5/1 -> Switch2/3
  Switch1/1 -> Add/1
  Switch/1 -> Add/2
  Switch2/1 -> Add/3
  Add/1 -> Multiport Switch/1

== system ZSM_TeslaModelS_statKreisfahrt/Vehicle/Betriebsstrategie/Momentenverteilung_und_Schaltstrategie1/Radmomentenaufteilung (Effizienz)/Umverteilung reduzieren ==
  note: Kein Sprung
  note: Umverteilung zwischen den Achsen
  note: Gangwechsel
  note: Pro Zeitschritt ein Prozent verändern
  note: Gangwechsel
  note: Sprünge von 0-100% ignorieren
  ind_unlim : Inport
  Abs : Abs
  Abs2 : Abs
  Add : Sum  Inputs=4
  Bias : Bias  Bias=-par_VEH.dt.ecu.n_Schaltkombinationen
  Bias1 : Bias  Bias=par_VEH.dt.ecu.n_Schaltkombinationen
  Compare To Constant1 : simulink/Logic and Bit Operations/Compare To Constant  relop=>=  const=(par_VEH.dt.ecu.Vektorlaenge*par_VEH.dt.ecu.n_Schaltkombinationen)-(4*par_VEH.dt.ecu.n_Schaltkombinationen)  OutDataTypeStr=boolean
  Compare To Constant2 : simulink/Logic and Bit Operations/Compare To Constant  relop=>=  const=par_VEH.dt.ecu.n_Schaltkombinationen  OutDataTypeStr=boolean
  Compare To Constant3 : simulink/Logic and Bit Operations/Compare To Constant  relop=<  const=par_VEH.dt.ecu.n_Schaltkombinationen  OutDataTypeStr=boolean
  Compare To Constant5 : simulink/Logic and Bit Operations/Compare To Constant  relop=>=  const=1  OutDataTypeStr=boolean
  Compare To Constant6 : simulink/Logic and Bit Operations/Compare To Constant  relop===  const=0  OutDataTypeStr=boolean
  Compare To Constant7 : simulink/Logic and Bit Operations/Compare To Constant  relop=<  const=(par_VEH.dt.ecu.Vektorlaenge*par_VEH.dt.ecu.n_Schaltkombinationen)-(4*par_VEH.dt.ecu.n_Schaltkombinationen)  OutDataTypeStr=boolean
  Constant : Constant  Value=par_VEH.dt.ecu.n_Schaltkombinationen
  Constant1 : Constant  Value=4
  Constant2 : Constant  Value=0
  Constant3 : Constant  Value=3
  Constant4 : Constant  Value=0
  Constant5 : Constant  Value=2
  Constant6 : Constant  Value=0
  Logical Operator : Logic  AllPortsSameDT=off  OutDataTypeStr=boolean
  Logical Operator2 : Logic  AllPortsSameDT=off  OutDataTypeStr=boolean
  Memory1 : Memory  InitialCondition=1
  Multiport Switch : MultiPortSwitch  Inputs=4
  Product : Product
  Relational Operator : RelationalOperator  Operator=<  OutDataTypeStr=boolean  RndMeth=Nearest
  Relational Operator1 : RelationalOperator  Operator=<  OutDataTypeStr=boolean  RndMeth=Nearest
  Schaltkombinationen : Constant  Value=par_VEH.dt.ecu.n_Schaltkombinationen
  Subtract : Sum  Inputs=+-
  Subtract2 : Sum  Inputs=+-
  Switch{,1..5} (6 alike) : Switch  Criteria=u2 > Threshold
  Vektorlänge : Constant  Value=par_VEH.dt.ecu.Vektorlaenge
  ind_lim : Outport  VectorParamsAs1DForOutWhenUnconnected=off
  wires:
  Switch2/1 -> Relational Operator/1, Switch1/1, Subtract/1
  Relational Operator/1 -> Switch/2
  Bias/1 -> Switch/1
  Bias1/1 -> Switch/3
  Relational Operator1/1 -> Switch1/2
  Switch1/1 -> Memory1/1, ind_lim/1
  Subtract/1 -> Abs/1
  Abs/1 -> Relational Operator1/1
  Constant/1 -> Relational Operator1/2
  Memory1/1 -> Switch2/3, Subtract/2, Relational Operator/2, Bias1/1, Bias/1, Subtract2/2
  Switch/1 -> Switch1/3
  Subtract2/1 -> Abs2/1
  Compare To Constant1/1 -> Logical Operator/1
  Compare To Constant2/1 -> Logical Operator/2
  Abs2/1 -> Compare To Constant7/1, Compare To Constant6/1, Compare To Constant5/1, Compare To Constant3/1, Compare To Constant2/1, Compare To Constant1/1
  Compare To Constant3/1 -> Logical Operator2/1
  Compare To Constant5/1 -> Logical Operator2/2
  Logical Operator2/1 -> Switch4/2
  Compare To Constant6/1 -> Switch3/2
  Add/1 -> Multiport Switch/1
  Constant1/1 -> Switch3/1
  Constant2/1 -> Switch3/3
  Switch3/1 -> Add/4
  Constant3/1 -> Switch4/1
  Constant4/1 -> Switch4/3
  Switch4/1 -> Add/3
  Logical Operator/1 -> Switch5/2
  Constant5/1 -> Switch5/1
  Constant6/1 -> Switch5/3
  Switch5/1 -> Add/2
  Compare To Constant7/1 -> Add/1, Switch2/2
  ind_unlim/1 -> Switch2/1, Subtract2/1
  Vektorlänge/1 -> Product/1
  Schaltkombinationen/1 -> Product/2

== system ZSM_TeslaModelS_statKreisfahrt/Vehicle/Betriebsstrategie/Momentenverteilung_und_Schaltstrategie1/Radmomentenaufteilung (Effizienz)/Vektorerstellung ==
  M_VA_pot : Inport
  M_HA_pot : Inport  Port=2
  M_wheel : Inport  Port=3
  Major_index_in : Inport  Port=4
  Constant : Constant  Value=ones(par_VEH.dt.ecu.n_Schaltkombinationen, 1)
  Product1 : Product
  Product2 : Product
  Product6 : Product  Multiplication=Matrix(*)
  Subtract1 : Sum  Inputs=-+
  Subtract2 : Sum  Inputs=+-
  Switch : Switch  Criteria=u2 > Threshold
  Switch1 : Switch  Criteria=u2 > Threshold
  Vektorerstellung : Constant  Value=0:par_VEH.dt.ecu.Vektorabstufung:1  VectorParams1D=off
  M_VA : Outport  VectorParamsAs1DForOutWhenUnconnected=off
  M_VA_pot_out : Outport  Port=2  VectorParamsAs1DForOutWhenUnconnected=off
  M_HA : Outport  Port=3  VectorParamsAs1DForOutWhenUnconnected=off
  M_HA_pot_out : Outport  Port=4  VectorParamsAs1DForOutWhenUnconnected=off
  Major_index_out : Outport  Port=5  VectorParamsAs1DForOutWhenUnconnected=off
  wires:
  Constant/1 -> Product6/1
  Vektorerstellung/1 -> Product6/2
  Product6/1 -> Product2/1, Product1/2  "M_VA"
  M_VA_pot/1 -> M_VA_pot_out/1, Product1/1
  Product1/1 -> Subtract1/1, Switch/1
  M_HA_pot/1 -> M_HA_pot_out/1, Product2/2
  Subtract1/1 -> Switch1/1
  M_wheel/1 -> Subtract2/1, Subtract1/2
  Switch/1 -> M_VA/1
  Major_index_in/1 -> Major_index_out/1, Switch1/2, Switch/2
  Product2/1 -> Switch1/3, Subtract2/2
  Subtract2/1 -> Switch/3
  Switch1/1 -> M_HA/1

== system ZSM_TeslaModelS_statKreisfahrt/Vehicle/Betriebsstrategie/Momentenverteilung_und_Schaltstrategie1/Radmomentenaufteilung (Effizienz)/Verlustleistung kann nicht Null sein ==
  Pv_GES_in : Inport
  Constant10 : Constant  Value=0
  Constant11 : Constant  Value=NaN
  Relational Operator1 : RelationalOperator  Operator===  OutDataTypeStr=boolean  RndMeth=Nearest
  Reshape : Reshape
  Switch : Switch  Criteria=u2 > Threshold
  Pv_GES_out : Outport  VectorParamsAs1DForOutWhenUnconnected=off
  wires:
  Constant11/1 -> Switch/1
  Constant10/1 -> Relational Operator1/1
  Switch/1 -> Reshape/1
  Pv_GES_in/1 -> Switch/3, Relational Operator1/2
  Reshape/1 -> Pv_GES_out/1
  Relational Operator1/1 -> Switch/2

== system ZSM_TeslaModelS_statKreisfahrt/Vehicle/Betriebsstrategie/Momentenverteilung_und_Schaltstrategie1/Radmomentenaufteilung (Standardfahrmanöver)/Limits ==
  Limits : Inport
  M_wheel : Inport  Port=2
  Add : Sum  Inputs=++++
  Bus Selector : BusSelector  OutputSignals=Fx_LF_ub,Fx_LF_lb,Fx_RF_ub,Fx_RF_lb,Fx_LR_ub,Fx_LR_lb,Fx_RR_ub,Fx_RR_lb
  Sign : Signum
  Switch{,1..3} (4 alike) : Switch
  X_Max : Outport  VectorParamsAs1DForOutWhenUnconnected=off
  Limit_FL : Outport  Port=2  VectorParamsAs1DForOutWhenUnconnected=off
  Limit_FR : Outport  Port=3  VectorParamsAs1DForOutWhenUnconnected=off
  Limit_RL : Outport  Port=4  VectorParamsAs1DForOutWhenUnconnected=off
  Limit_RR : Outport  Port=5  VectorParamsAs1DForOutWhenUnconnected=off
  wires:
  Limits/1 -> Bus Selector/1
  M_wheel/1 -> Sign/1
  Bus Selector/1 -> Switch/1  "<Fx_LF_ub>"
  Bus Selector/2 -> Switch/3  "<Fx_LF_lb>"
  Bus Selector/3 -> Switch1/1  "<Fx_RF_ub>"
  Bus Selector/4 -> Switch1/3  "<Fx_RF_lb>"
  Bus Selector/5 -> Switch2/1  "<Fx_LR_ub>"
  Bus Selector/6 -> Switch2/3  "<Fx_LR_lb>"
  Bus Selector/7 -> Switch3/1  "<Fx_RR_ub>"
  Bus Selector/8 -> Switch3/3  "<Fx_RR_lb>"
  Sign/1 -> Switch/2, Switch1/2, Switch2/2, Switch3/2
  Add/1 -> X_Max/1
  Switch3/1 -> Add/4, Limit_RR/1
  Switch2/1 -> Add/3, Limit_RL/1
  Switch1/1 -> Add/2, Limit_FR/1
  Switch/1 -> Add/1, Limit_FL/1

== system ZSM_TeslaModelS_statKreisfahrt/Vehicle/Betriebsstrategie/Momentenverteilung_und_Schaltstrategie1/Radmomentenaufteilung (Standardfahrmanöver)/MomentForce ==
  Input : Inport
  MWheel : Inport  Port=2
  Add : Sum  Inputs=++++
  Bus Selector : BusSelector  OutputSignals=r_stat.r_stat_RF,r_stat.r_stat_LF,r_stat.r_stat_RR,r_stat.r_stat_LR
  Divide : Product  Inputs=*/
  Gain : Gain  Gain=1/4
  IC : InitialCondition  Value=par_VEH.r_stat0
  XWheel : Outport  VectorParamsAs1DForOutWhenUnconnected=off
  wires:
  MWheel/1 -> Divide/1
  Input/1 -> Bus Selector/1
  Bus Selector/1 -> Add/1  "<r_stat_RF>"
  Bus Selector/2 -> Add/2  "<r_stat_LF>"
  Bus Selector/3 -> Add/3  "<r_stat_RR>"
  Bus Selector/4 -> Add/4  "<r_stat_LR>"
  Add/1 -> Gain/1
  Divide/1 -> XWheel/1
  Gain/1 -> IC/1
  IC/1 -> Divide/2

== system ZSM_TeslaModelS_statKreisfahrt/Vehicle/Betriebsstrategie/Momentenverteilung_und_Schaltstrategie1/Radmomentenaufteilung (Standardfahrmanöver)/MomentForce1 ==
  Fx_RF : Inport
  Fx_LF : Inport  Port=2
  Fx_RR : Inport  Port=3
  Fx_LR : Inport  Port=4
  Input : Inport  Port=5
  Bus Selector : BusSelector  OutputSignals=r_stat.r_stat_RF,r_stat.r_stat_LF,r_stat.r_stat_RR,r_stat.r_stat_LR
  IC{,1..3} (4 alike) : InitialCondition  Value=par_VEH.r_stat0
  Product{,1..3} (4 alike) : Product
  M_antr_RF : Outport  VectorParamsAs1DForOutWhenUnconnected=off
  M_antr_LF : Outport  Port=2  VectorParamsAs1DForOutWhenUnconnected=off
  M_antr_RR : Outport  Port=3  VectorParamsAs1DForOutWhenUnconnected=off
  M_antr_LR : Outport  Port=4  VectorParamsAs1DForOutWhenUnconnected=off
  wires:
  Input/1 -> Bus Selector/1
  Bus Selector/1 -> IC/1  "<r_stat_RF>"
  Bus Selector/2 -> IC1/1  "<r_stat_LF>"
  Bus Selector/3 -> IC2/1  "<r_stat_RR>"
  Bus Selector/4 -> IC3/1  "<r_stat_LR>"
  Product/1 -> M_antr_RF/1
  Fx_RF/1 -> Product/2
  Fx_LF/1 -> Product1/2
  Fx_RR/1 -> Product2/2
  Fx_LR/1 -> Product3/2
  Product1/1 -> M_antr_LF/1
  Product2/1 -> M_antr_RR/1
  Product3/1 -> M_antr_LR/1
  IC/1 -> Product/1
  IC1/1 -> Product1/1
  IC2/1 -> Product2/1
  IC3/1 -> Product3/1
